simulink model "BatterySoC"  (R2020a)
settings: Solver=VariableStepAuto  StartTime=0.0  StopTime=550  RelTol=1e-3
undefined symbols (not defined in the file or in its folder): DiscIntNeverNeededParam, Ion, Lithium
libraries: powerlib x11, electricdrivelib x1
settings Model: Creator=bolt  LastModifiedBy=Marvin

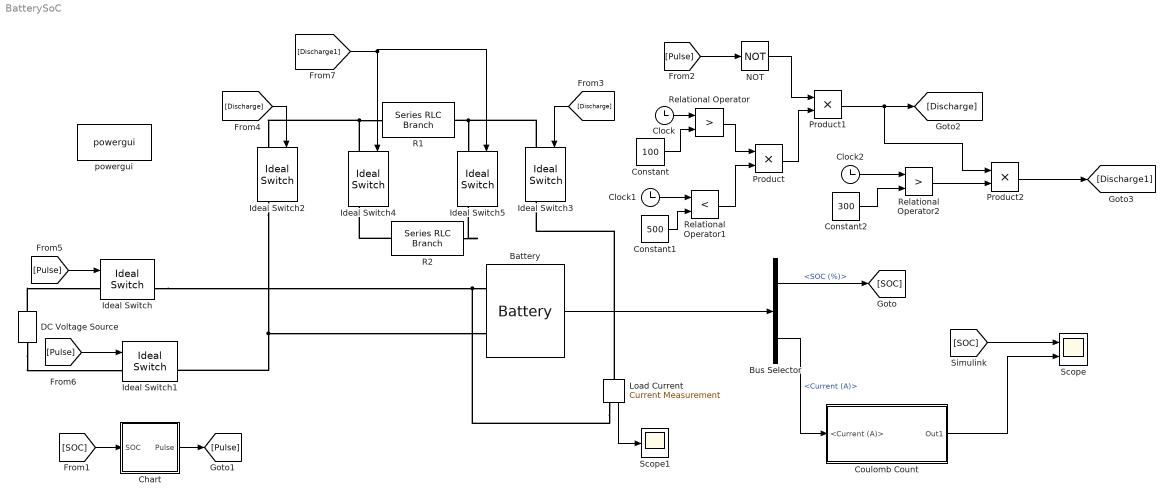
== system BatterySoC ==
  Battery : electricdrivelib/Extra Sources/Battery  BatType=Lithium-Ion  ShowTempParam=off  ThermalPreset=no  ShowAgeParam=off  NomV=3.7  NomQ=1.5  SOC=30  Batt_Tr=1  PresetModel=on  MaxQ=1.5  MinV=2.775  FullV=4.3068  Dis_rate=0.65217  R=0.024667  Normal_OP=1.3565  expZone="[3.9974    0.073696]"  current=[6.5 13 32.5]  Units=Time  Tci=20  NomT=20  T2=-30  MaxQ2=4.8  FullV2=7.1  Normal_OP2=5.655  expZone2="[6.58           1]"  Rca=0.6  ti=2000  Dp=0  Neq0=0  Tsim=1e6  Ta1=25  Qeol=5.4*0.9  Reol=0.013333*1.2  Char_age=[2.3478, 3]  Dis_age=[2.3478, 10]  N1=1500  N2=10500  N3=1000  N4=1400  Ta2=45  N5=950
  Bus Selector : BusSelector  OutputSignals=SOC (%),Current (A)
  Chart : Stateflow chart  TreatAsAtomicUnit=on
  Clock : Clock
  Clock1 : Clock
  Clock2 : Clock
  Constant : Constant  Value=100
  Constant1 : Constant  Value=500
  Constant2 : Constant  Value=300
  Coulomb Count : Subsystem
  DC Voltage Source : powerlib/Electrical Sources/DC Voltage Source  Amplitude=9  Measurements=None
  Ideal Switch{,1..5} (6 alike) : powerlib/Power Electronics/Ideal Switch  Ron=0.001  Lon=0  IC=0  Rs=1e5  Cs=inf  Measurements=on
  Load Current : powerlib/Measurements/Current Measurement  PhasorSimulation=off  OutputType=Complex  PSBequivalent=0
  NOT : Logic  Operator=NOT  IconShape=distinctive  AllPortsSameDT=off  OutDataTypeStr=boolean
  Product : Product
  Product1 : Product
  Product2 : Product
  R1 : powerlib/Elements/Series RLC Branch  LConnTagsString=__new0  RConnTagsString=__new0  BranchType=R  Resistance=0.84  Inductance=1e-3  SetiL0=off  InitialCurrent=0  Capacitance=1e-6  Setx0=off  InitialVoltage=0  Measurements=None
  R2 : powerlib/Elements/Series RLC Branch  LConnTagsString=__new0  RConnTagsString=__new0  BranchType=R  Resistance=0.68  Inductance=1e-3  SetiL0=off  InitialCurrent=0  Capacitance=1e-6  Setx0=off  InitialVoltage=0  Measurements=None
  Relational Operator : RelationalOperator  Operator=>  OutDataTypeStr=boolean  RndMeth=Simplest
  Relational Operator1 : RelationalOperator  Operator=<  OutDataTypeStr=boolean  RndMeth=Simplest
  Relational Operator2 : RelationalOperator  Operator=>  OutDataTypeStr=boolean  RndMeth=Simplest
  Scope : Scope  NumInputPorts=2
  Scope1 : Scope
  powergui : powerlib/powergui  Priority=1  SimulationMode=Discrete  SampleTime=50e-4  frequency=60  Iterations=50  frequencyindice=0  Pbase=100e6  ErrMax=1e-4  UnitsV=kV  UnitsW=MW  buscounter=0  FunctionMessages=off  echomessages=off  EnableUseOfTLC=off  CurrentSourceSwitches=off  DisableSnubberDevices=off  DisableRonSwitches=off  DisableVfSwitches=off  DisplayEquations=off  AutomaticDiscreteSolvers=off  SolverType=Tustin/Backward Euler (TBE)  Interpol=off  ExternalGateDelay=off  methode=off  Ts=100  x0status=blocks  SPID=on  SwTol=0  HookPort=off  NonlinearTolerance=1e-4  nMaxIteration=100  ContinueOnMaxIteration=off  RestoreLinks=warning  ResistiveCurrentMeasurement=off  Frange=[0:2:500]  Ylog=off  Xlog=on  ShowGrid=off  save=off  variable=ZData  structure=0  ZoomFFT=off  StartTime=0.0  cycles=1  DisplayStyle=1  fundamental=60  FreqAxis=off  MaxFrequency=1000  frequencyindicesteady=1  RmsSteady=1  display=off
  wires:
  Battery/1 -> Bus Selector/1
  Bus Selector/1 -> [SOC]  "<SOC (%)>"
  [SOC] -> Scope/1
  [SOC] -> Chart/1(SOC)
  Chart/1(Pulse) -> [Pulse]
  [Discharge] -> Ideal Switch2/1
  [Discharge] -> Ideal Switch3/1
  [Pulse] -> Ideal Switch/1
  [Pulse] -> Ideal Switch1/1
  Bus Selector/2 -> Coulomb Count/1(<Current (A)>)  "<Current (A)>"
  Coulomb Count/1(Out1) -> Scope/2
  [Discharge1] -> Ideal Switch5/1, Ideal Switch4/1
  Product1/1 -> Product2/1, [Discharge]
  Clock/1 -> Relational Operator/1
  Clock1/1 -> Relational Operator1/1
  Constant1/1 -> Relational Operator1/2
  Relational Operator2/1 -> Product2/2
  Product2/1 -> [Discharge1]
  NOT/1 -> Product1/1
  Constant/1 -> Relational Operator/2
  Clock2/1 -> Relational Operator2/1
  Constant2/1 -> Relational Operator2/2
  [Pulse] -> NOT/1
  Relational Operator1/1 -> Product/2
  Relational Operator/1 -> Product/1
  Product/1 -> Product1/2
  Load Current/1 -> Scope1/1
  connections:
  DC Voltage Source/LConn1 -- Ideal Switch/LConn1
  Ideal Switch/RConn1 -- Load Current/RConn1 -- Battery/LConn2
  DC Voltage Source/RConn1 -- Ideal Switch1/LConn1
  Ideal Switch4/LConn1 -- R1/LConn1 -- Ideal Switch2/LConn1
  Ideal Switch2/RConn1 -- Ideal Switch1/RConn1 -- Battery/LConn1
  Ideal Switch3/LConn1 -- R1/RConn1 -- Ideal Switch5/LConn1
  R2/RConn1 -- Ideal Switch5/RConn1
  R2/LConn1 -- Ideal Switch4/RConn1
  Load Current/LConn1 -- Ideal Switch3/RConn1

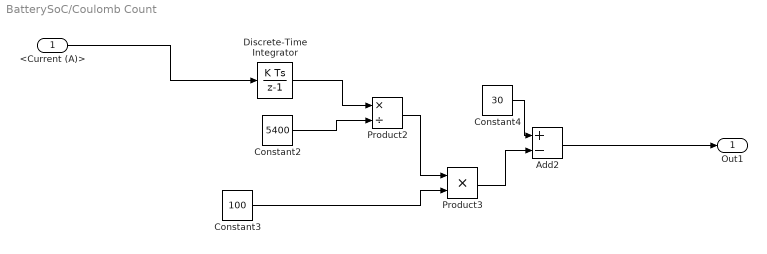
== system BatterySoC/Coulomb Count ==
  <Current (A)> : Inport
  Add2 : Sum  Inputs=+-
  Constant2 : Constant  Value=5400
  Constant3 : Constant  Value=100
  Constant4 : Constant  Value=30
  Discrete-Time Integrator : DiscreteIntegrator  gainval=1  SampleTime=-1  LimitOutput=on  UpperSaturationLimit=100  ICPrevOutput=DiscIntNeverNeededParam  ICPrevScaledInput=DiscIntNeverNeededParam
  Product2 : Product  Inputs=*/
  Product3 : Product
  Out1 : Outport
  wires:
  <Current (A)>/1 -> Discrete-Time Integrator/1
  Constant4/1 -> Add2/1
  Add2/1 -> Out1/1
  Constant2/1 -> Product2/2
  Discrete-Time Integrator/1 -> Product2/1
  Constant3/1 -> Product3/2
  Product2/1 -> Product3/1
  Product3/1 -> Add2/2

== stateflow chart BatterySoC/Chart ==
  state Charge
    entry : Pulse =1
  state Discharge
    entry : Pulse = 0
  (default) -> Charge
  Charge -> Discharge : [SOC>99.99]
  Discharge -> Charge : [SOC<30]
  data: SOC input; Pulse output
